simulink model "EJ3_2_2_Simulink"  (R2014a)
settings: Solver=ode45  StartTime=0.0  StopTime=10.0  RelTol=1e-3
undefined symbols (not defined in the file or in its folder): den1, den2, den3, num1, num2, num3
settings Model: Creator=sebar  LastModifiedBy=sebar

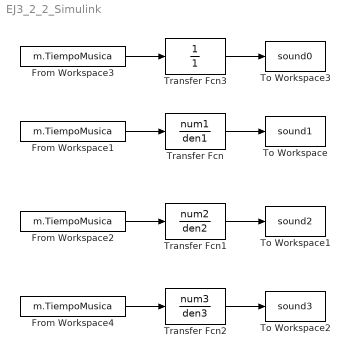
== system EJ3_2_2_Simulink ==
  From Workspace{1..4} (4 alike) : FromWorkspace  VariableName=m.TiempoMusica  SampleTime=0
  To Workspace : ToWorkspace  VariableName=sound1  SaveFormat=Timeseries  SampleTime=1/11025
  To Workspace1 : ToWorkspace  VariableName=sound2  SaveFormat=Timeseries  SampleTime=1/11025
  To Workspace2 : ToWorkspace  VariableName=sound3  SaveFormat=Timeseries  SampleTime=1/11025
  To Workspace3 : ToWorkspace  VariableName=sound0  SaveFormat=Timeseries  SampleTime=1/11025
  Transfer Fcn : TransferFcn  Numerator=num1  Denominator=den1
  Transfer Fcn1 : TransferFcn  Numerator=num2  Denominator=den2
  Transfer Fcn2 : TransferFcn  Numerator=num3  Denominator=den3
  Transfer Fcn3 : TransferFcn  Numerator=1  Denominator=1
  wires:
  From Workspace1/1 -> Transfer Fcn/1
  Transfer Fcn/1 -> To Workspace/1
  From Workspace2/1 -> Transfer Fcn1/1
  Transfer Fcn1/1 -> To Workspace1/1
  From Workspace4/1 -> Transfer Fcn2/1
  Transfer Fcn2/1 -> To Workspace2/1
  From Workspace3/1 -> Transfer Fcn3/1
  Transfer Fcn3/1 -> To Workspace3/1
